simulink subsystem "residueAmplifier"  (R2024b)
settings: Solver=VariableStepAuto  StartTime=0.0  StopTime=10.0  RelTol=1e-3
values from neighbouring files (symbols this model uses):
  C_f1 = C_s/G1    (= 2.5e-10)    [TestWrapper.m]
  C_s = 2000000e-15    (= 2e-09)    [TestWrapper.m]
  G1 = 2^(B1-1)    (= 8)    [TestWrapper.m]
  k = 1.38e-23    [TestWrapper.m]
  LGBW = 30*fs    (= 9000000000)    [TestWrapper.m]
  T = 300    [TestWrapper.m]
  ts = 1/fs    (= 3.33333333333e-09)    [TestWrapper.m]
libraries: dspsrcs4 x1
settings Model: Creator=bbassett6  LastModifiedBy=bbassett6

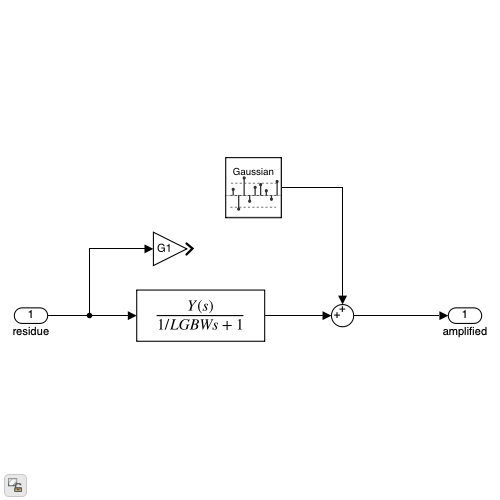
[thumbnail: Simulink's stored preview of the top-level diagram]
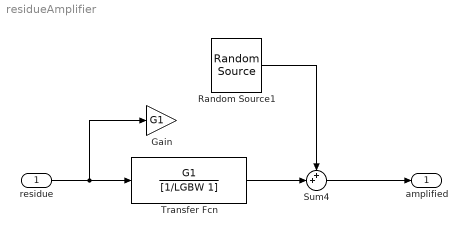
== system residueAmplifier ==
  residue : Inport
  Gain : Gain  Gain=G1
  Random Source1 : dspsrcs4/Random Source  SrcType=Gaussian  MinVal=0  MaxVal=1  MeanVal=0  VarVal=2*k*T*(C_s+C_f1)/C_f1^2  RepMode=Not repeatable  rawSeed=1  IsInherit=off  SampTime=ts/2  SampFrame=1  OutComplex=Real  DataType=double  SimulateUsing=Interpreted execution
  Sum4 : Sum  Inputs=++|
  Transfer Fcn : TransferFcn  Numerator=G1  Denominator=[1/LGBW 1]
  amplified : Outport
  wires:
  Sum4/1 -> amplified/1
  residue/1 -> Gain/1, Transfer Fcn/1
  Random Source1/1 -> Sum4/1
  Transfer Fcn/1 -> Sum4/2
